simulink model "f7_VPP_DER_demo"  (R2019b)
settings: Solver=VariableStepAuto  StartTime=0.0  StopTime=2  FixedStep=1e-9  RelTol=1e-2
PreLoadFcn:
  | ss=2;sr=0;
InitFcn:
  | ss=2;sr=0;
libraries: powerlib x35, powerlib_meascontrol x30
settings Model: SimulationMode=accelerator  Creator=MAHMUD  LastModifiedBy=MAHMUD
settings SolverCC: ZeroCrossAlgorithm=Adaptive
settings DataIOCC: ReturnWorkspaceOutputs=off
settings DebuggingCC: MaxConsecutiveZCsMsg=none  IgnoredZcDiagnostic=none  ArithmeticOperatorsInVariantConditions=warning
settings SFSimCC: SimUseLocalCustomCode=off  CustomCodeUndefinedFunction=UseInterfaceOnly
settings RTWCC: RTWUseLocalCustomCode=off

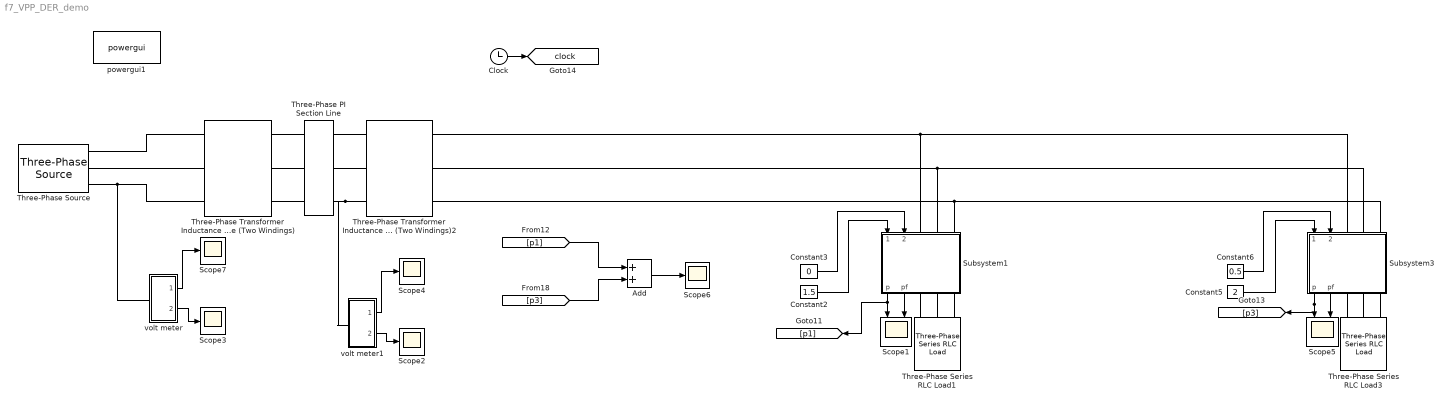
== system f7_VPP_DER_demo ==
  Add : Sum  Inputs=2
  Clock : Clock
  Constant2 : Constant  Value=1.5
  Constant3 : Constant  Value=0
  Constant5 : Constant  Value=2
  Constant6 : Constant  Value=0.5
  Scope1 : Scope  NumInputPorts=2
  Scope{2..4,6..7} (5 alike) : Scope
  Scope5 : Scope  NumInputPorts=2
  Subsystem1 : Subsystem
  Subsystem3 : Subsystem
  Three-Phase PI Section Line : powerlib/Elements/Three-Phase PI Section Line  LConnTagsString=a|b|c  RConnTagsString=A|B|C  Frequency=50  Resistances=[ 0.01273 0.3864]  Inductances="[ 0.9337e-3  4.1264e-3]"  Capacitances=[12.74e-9 7.751e-9]  Length=100
      settings: SourceProductName=Simscape Electrical
  Three-Phase Series RLC Load1 : powerlib/Elements/Three-Phase Series RLC Load  LConnTagsString=A|B|C  Configuration=Y (grounded)  NominalVoltage=240  Vabc=[240 240 240]  Vabcp=[1e3 1e3 1e3]  NominalFrequency=50  UnbalancedPower=off  ActivePower=5e3  InductivePower=0  CapacitivePower=0  Pabc=[10e3 9e3 11e3]  QLabc=[100 90 110]  QCabc=[100 90 110]  Pabcp=[10e3 9e3 11e3]  QLabcp=[100 90 110]  QCabcp=[100 90 110]  Measurements=None  LoadType=constant PQ
      settings: SourceProductName=Simscape Electrical
  Three-Phase Series RLC Load3 : powerlib/Elements/Three-Phase Series RLC Load  LConnTagsString=A|B|C  Configuration=Y (grounded)  NominalVoltage=240  Vabc=[1e3 1e3 1e3]  Vabcp=[1e3 1e3 1e3]  NominalFrequency=50  UnbalancedPower=off  ActivePower=2e3  InductivePower=5e3  CapacitivePower=0  Pabc=[10e3 9e3 11e3]  QLabc=[100 90 110]  QCabc=[100 90 110]  Pabcp=[10e3 9e3 11e3]  QLabcp=[100 90 110]  QCabcp=[100 90 110]  Measurements=None  LoadType=constant PQ
      settings: SourceProductName=Simscape Electrical
  Three-Phase Source : powerlib/Electrical Sources/Three-Phase Source  InternalConnection=Yg  VoltagePhases=off  Voltage=14270  PhaseAngle=0  Voltage_phases=[25e3 25e3 25e3]/sqrt(3)  PhaseAngles_phases=[0 -120 +120]  Frequency=50  NonIdealSource=on  SpecifyImpedance=off  Resistance=0.8929  Inductance=0  ShortCircuitLevel=100e6  BaseVoltage=15000  XRratio=7  BusType=PQ  Pref=30e3  Qref=0  Prefabc=[10e3, 10e3, 10e3]  Qrefabc=[0, 0, 0]  Qmin=-inf  Qmax=inf
      settings: SourceProductName=Simscape Electrical
  Three-Phase Transformer Inductance Matrix Type (Two Windings) : powerlib/Elements/Three-Phase Transformer Inductance Matrix Type (Two Windings)  CoreType=Three-limb or five-limb core  Winding1Connection=Yg  Winding2Connection=Yg  AutoTransformer=off  Measurements=None  NominalPower=[100e3, 50]  VLLnom=[25000, 130000]  WindingResistances=[0.01, 0.01]  NoLoadIexcPos=2  NoLoadPlossPos=1000  ShortCircuitReactancePos=0.06  ShortCircuitReactancePosAuto=0.06  NoLoadIexcZero=100  NoLoadPlossZero=1500  ShortCircuitReactanceZero=0.03  ShortCircuitReactanceZeroAuto=0.03
      settings: SourceProductName=Simscape Electrical  SourceProductBaseCode=PS
  Three-Phase Transformer Inductance Matrix Type (Two Windings)2 : powerlib/Elements/Three-Phase Transformer Inductance Matrix Type (Two Windings)  CoreType=Three-limb or five-limb core  Winding1Connection=Yg  Winding2Connection=Yg  AutoTransformer=off  Measurements=None  NominalPower=[30e3, 50]  VLLnom=[12700, 240]  WindingResistances=[0.01, 0.01]  NoLoadIexcPos=4  NoLoadPlossPos=1000  ShortCircuitReactancePos=0.06  ShortCircuitReactancePosAuto=0.06  NoLoadIexcZero=100  NoLoadPlossZero=1500  ShortCircuitReactanceZero=0.03  ShortCircuitReactanceZeroAuto=0.03
      settings: SourceProductName=Simscape Electrical  SourceProductBaseCode=PS
  powergui1 : powerlib/powergui  Priority=1  SimulationMode=Continuous  SampleTime=50e-6  frequency=60  Iterations=50  frequencyindice=50  Pbase=100e6  ErrMax=1e-4  UnitsV=kV  UnitsW=MW  buscounter=0  FunctionMessages=off  echomessages=off  EnableUseOfTLC=off  CurrentSourceSwitches=off  DisableSnubberDevices=off  DisableRonSwitches=off  DisableVfSwitches=off  DisplayEquations=off  AutomaticDiscreteSolvers=off  SolverType=Tustin/Backward Euler (TBE)  Interpol=off  ExternalGateDelay=off  methode=off  Ts=100  x0status=blocks  SPID=on  SwTol=0  HookPort=off  NonlinearTolerance=1e-4  nMaxIteration=100  ContinueOnMaxIteration=off  RestoreLinks=warning  ResistiveCurrentMeasurement=off  Frange=[0:2:500]  Ylog=off  Xlog=on  ShowGrid=off  save=off  variable=ZData  structure=0  ZoomFFT=off  StartTime=0.0  cycles=1  DisplayStyle=1  fundamental=60  FreqAxis=off  MaxFrequency=1000  frequencyindicesteady=1  RmsSteady=1  display=off
      settings: SourceProductName=Simscape Electrical
  volt meter : Subsystem
  volt meter1 : Subsystem
  tag scope: clock=global
  wires:
  Subsystem3/2(pf) -> Scope5/2
  Constant2/1 -> Subsystem1/1(stop time)
  volt meter1/2(Vrms) -> Scope2/1
  [p1] -> Add/1
  Constant3/1 -> Subsystem1/2(start time)
  Subsystem1/1(p) -> [p1], Scope1/1
  Subsystem1/2(pf) -> Scope1/2
  volt meter/1(Vsin) -> Scope7/1
  volt meter1/1(Vsin) -> Scope4/1
  volt meter/2(Vrms) -> Scope3/1
  Constant5/1 -> Subsystem3/1(stop time)
  Subsystem3/1(p) -> [p3], Scope5/1
  Constant6/1 -> Subsystem3/2(start time)
  [p3] -> Add/2
  Clock/1 -> [clock]
  Add/1 -> Scope6/1
  connections:
  Subsystem1/LConn2 -- Three-Phase Transformer Inductance Matrix Type (Two Windings)2/RConn2 -- Subsystem3/LConn2
  Three-Phase Transformer Inductance Matrix Type (Two Windings)/LConn3 -- Three-Phase Source/RConn3 -- volt meter/LConn1
  Subsystem1/LConn3 -- Three-Phase Transformer Inductance Matrix Type (Two Windings)2/RConn3 -- Subsystem3/LConn3
  Subsystem1/LConn1 -- Three-Phase Transformer Inductance Matrix Type (Two Windings)2/RConn1 -- Subsystem3/LConn1
  Three-Phase Transformer Inductance Matrix Type (Two Windings)2/LConn3 -- Three-Phase PI Section Line/RConn3 -- volt meter1/LConn1
  Subsystem3/RConn3 -- Three-Phase Series RLC Load3/LConn3
  Three-Phase Transformer Inductance Matrix Type (Two Windings)/RConn3 -- Three-Phase PI Section Line/LConn3
  Subsystem3/RConn1 -- Three-Phase Series RLC Load3/LConn1
  Three-Phase PI Section Line/RConn2 -- Three-Phase Transformer Inductance Matrix Type (Two Windings)2/LConn2
  Three-Phase PI Section Line/LConn1 -- Three-Phase Transformer Inductance Matrix Type (Two Windings)/RConn1
  Three-Phase Source/RConn1 -- Three-Phase Transformer Inductance Matrix Type (Two Windings)/LConn1
  Subsystem1/RConn2 -- Three-Phase Series RLC Load1/LConn2
  Subsystem1/RConn3 -- Three-Phase Series RLC Load1/LConn3
  Three-Phase PI Section Line/LConn2 -- Three-Phase Transformer Inductance Matrix Type (Two Windings)/RConn2
  Subsystem1/RConn1 -- Three-Phase Series RLC Load1/LConn1
  Three-Phase Source/RConn2 -- Three-Phase Transformer Inductance Matrix Type (Two Windings)/LConn2
  Three-Phase Transformer Inductance Matrix Type (Two Windings)2/LConn1 -- Three-Phase PI Section Line/RConn1
  Subsystem3/RConn2 -- Three-Phase Series RLC Load3/LConn2

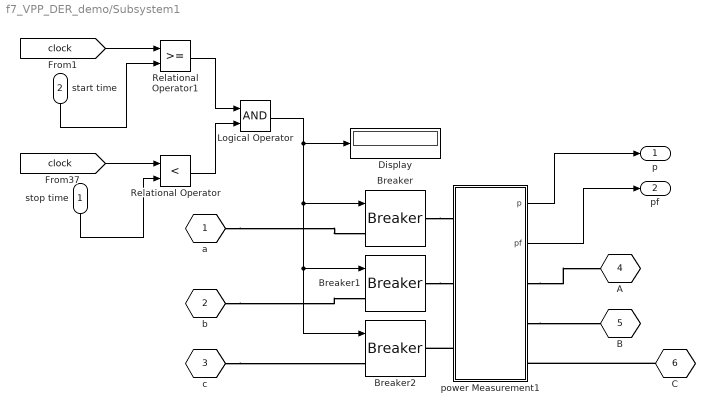
== system f7_VPP_DER_demo/Subsystem1 ==
  stop time : Inport
  start time : Inport  Port=2
  Breaker : powerlib/Elements/Breaker  InitialState=0  SwitchingTimes="[1/60  5/60]"  External=on  BreakerResistance=0.01  SnubberResistance=1e6  SnubberCapacitance=inf  Measurements=None  MoreParameters=on  NoBreakLoop=off
      settings: SourceProductName=Simscape Electrical
  Breaker1 : powerlib/Elements/Breaker  InitialState=0  SwitchingTimes="[1/60  5/60]"  External=on  BreakerResistance=0.01  SnubberResistance=1e6  SnubberCapacitance=inf  Measurements=None  MoreParameters=on  NoBreakLoop=off
      settings: SourceProductName=Simscape Electrical
  Breaker2 : powerlib/Elements/Breaker  InitialState=0  SwitchingTimes="[1/60  5/60]"  External=on  BreakerResistance=0.01  SnubberResistance=1e6  SnubberCapacitance=inf  Measurements=None  MoreParameters=on  NoBreakLoop=off
      settings: SourceProductName=Simscape Electrical
  Display : Display
  Logical Operator : Logic  AllPortsSameDT=off  OutDataTypeStr=boolean
  Relational Operator : RelationalOperator  Operator=<  OutDataTypeStr=boolean  ZeroCross=off  RndMeth=Simplest
  Relational Operator1 : RelationalOperator  OutDataTypeStr=boolean  ZeroCross=off  RndMeth=Simplest
  power Measurement1 : Subsystem
  a : PMIOPort  Tag=PMCPort  Side=Left
  b : PMIOPort  Tag=PMCPort  Port=2  Side=Left
  c : PMIOPort  Tag=PMCPort  Port=3  Side=Left
  "A " : PMIOPort  Tag=PMCPort  Port=4  Side=Right
  B : PMIOPort  Tag=PMCPort  Port=5  Side=Right
  C : PMIOPort  Tag=PMCPort  Port=6  Side=Right
  p : Outport
  pf : Outport  Port=2
  wires:
  Logical Operator/1 -> Breaker/1, Breaker2/1, Breaker1/1, Display/1
  [clock] -> Relational Operator/1
  stop time/1 -> Relational Operator/2
  [clock] -> Relational Operator1/1
  start time/1 -> Relational Operator1/2
  Relational Operator1/1 -> Logical Operator/1
  Relational Operator/1 -> Logical Operator/2
  power Measurement1/2(pf) -> pf/1
  power Measurement1/1(p) -> p/1
  connections:
  b/RConn1 -- Breaker1/LConn1
  c/RConn1 -- Breaker2/LConn1
  a/RConn1 -- Breaker/LConn1
  power Measurement1/RConn2 -- B/RConn1
  power Measurement1/LConn3 -- Breaker2/RConn1
  Breaker1/RConn1 -- power Measurement1/LConn2
  Breaker/RConn1 -- power Measurement1/LConn1
  C/RConn1 -- power Measurement1/RConn3
  power Measurement1/RConn1 -- "A "/RConn1

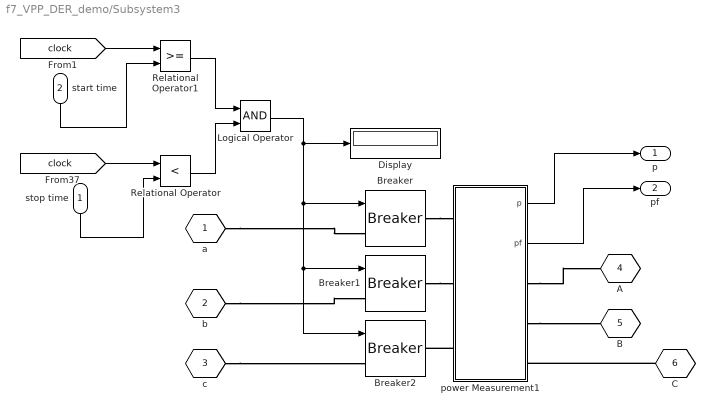
== system f7_VPP_DER_demo/Subsystem3 ==
  stop time : Inport
  start time : Inport  Port=2
  Breaker : powerlib/Elements/Breaker  InitialState=0  SwitchingTimes="[1/60  5/60]"  External=on  BreakerResistance=0.01  SnubberResistance=1e6  SnubberCapacitance=inf  Measurements=None  MoreParameters=on  NoBreakLoop=off
      settings: SourceProductName=Simscape Electrical
  Breaker1 : powerlib/Elements/Breaker  InitialState=0  SwitchingTimes="[1/60  5/60]"  External=on  BreakerResistance=0.01  SnubberResistance=1e6  SnubberCapacitance=inf  Measurements=None  MoreParameters=on  NoBreakLoop=off
      settings: SourceProductName=Simscape Electrical
  Breaker2 : powerlib/Elements/Breaker  InitialState=0  SwitchingTimes="[1/60  5/60]"  External=on  BreakerResistance=0.01  SnubberResistance=1e6  SnubberCapacitance=inf  Measurements=None  MoreParameters=on  NoBreakLoop=off
      settings: SourceProductName=Simscape Electrical
  Display : Display
  Logical Operator : Logic  AllPortsSameDT=off  OutDataTypeStr=boolean
  Relational Operator : RelationalOperator  Operator=<  OutDataTypeStr=boolean  ZeroCross=off  RndMeth=Simplest
  Relational Operator1 : RelationalOperator  OutDataTypeStr=boolean  ZeroCross=off  RndMeth=Simplest
  power Measurement1 : Subsystem
  a : PMIOPort  Tag=PMCPort  Side=Left
  b : PMIOPort  Tag=PMCPort  Port=2  Side=Left
  c : PMIOPort  Tag=PMCPort  Port=3  Side=Left
  "A " : PMIOPort  Tag=PMCPort  Port=4  Side=Right
  B : PMIOPort  Tag=PMCPort  Port=5  Side=Right
  C : PMIOPort  Tag=PMCPort  Port=6  Side=Right
  p : Outport
  pf : Outport  Port=2
  wires:
  Logical Operator/1 -> Breaker/1, Breaker2/1, Breaker1/1, Display/1
  [clock] -> Relational Operator/1
  stop time/1 -> Relational Operator/2
  [clock] -> Relational Operator1/1
  start time/1 -> Relational Operator1/2
  Relational Operator1/1 -> Logical Operator/1
  Relational Operator/1 -> Logical Operator/2
  power Measurement1/2(pf) -> pf/1
  power Measurement1/1(p) -> p/1
  connections:
  b/RConn1 -- Breaker1/LConn1
  c/RConn1 -- Breaker2/LConn1
  a/RConn1 -- Breaker/LConn1
  power Measurement1/RConn2 -- B/RConn1
  power Measurement1/LConn3 -- Breaker2/RConn1
  Breaker1/RConn1 -- power Measurement1/LConn2
  Breaker/RConn1 -- power Measurement1/LConn1
  C/RConn1 -- power Measurement1/RConn3
  power Measurement1/RConn1 -- "A "/RConn1

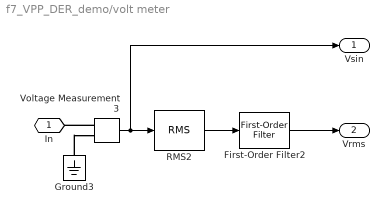
== system f7_VPP_DER_demo/volt meter ==
  First-Order Filter2 : powerlib_meascontrol/Filters/First-Order Filter  FilterType=Lowpass  Tc=100e-3  Ts=0  Initialize=off  Vac_Init=[0, 0, 50]  Vdc_Init=0  PlotResponse=off  FreqRange="[0,  200,  1]"
      settings: SourceProductName=Simscape Electrical
  Ground3 : powerlib/Elements/Ground  LConnTagsString=a
      settings: SourceProductName=Simscape Electrical
  RMS2 : powerlib_meascontrol/Measurements/RMS  TrueRMS=on  Freq=50  RMSInit=210  Ts=0.001
      settings: SourceProductName=Simscape Electrical
  Voltage Measurement3 : powerlib/Measurements/Voltage Measurement  PhasorSimulation=off  OutputType=Complex  PSBequivalent=0
      settings: SourceProductName=Simscape Electrical
  In : PMIOPort  Side=Left
  Vsin : Outport
  Vrms : Outport  Port=2
  wires:
  Voltage Measurement3/1 -> Vsin/1, RMS2/1
  RMS2/1 -> First-Order Filter2/1
  First-Order Filter2/1 -> Vrms/1
  connections:
  Ground3/LConn1 -- Voltage Measurement3/LConn2
  Voltage Measurement3/LConn1 -- In/RConn1

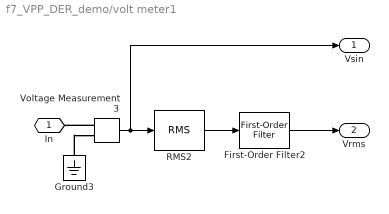
== system f7_VPP_DER_demo/volt meter1 ==
  First-Order Filter2 : powerlib_meascontrol/Filters/First-Order Filter  FilterType=Lowpass  Tc=100e-3  Ts=0  Initialize=off  Vac_Init=[0, 0, 50]  Vdc_Init=0  PlotResponse=off  FreqRange="[0,  200,  1]"
      settings: SourceProductName=Simscape Electrical
  Ground3 : powerlib/Elements/Ground  LConnTagsString=a
      settings: SourceProductName=Simscape Electrical
  RMS2 : powerlib_meascontrol/Measurements/RMS  TrueRMS=on  Freq=50  RMSInit=210  Ts=0.001
      settings: SourceProductName=Simscape Electrical
  Voltage Measurement3 : powerlib/Measurements/Voltage Measurement  PhasorSimulation=off  OutputType=Complex  PSBequivalent=0
      settings: SourceProductName=Simscape Electrical
  In : PMIOPort  Side=Left
  Vsin : Outport
  Vrms : Outport  Port=2
  wires:
  First-Order Filter2/1 -> Vrms/1
  RMS2/1 -> First-Order Filter2/1
  Voltage Measurement3/1 -> RMS2/1, Vsin/1
  connections:
  Voltage Measurement3/LConn1 -- In/RConn1
  Ground3/LConn1 -- Voltage Measurement3/LConn2

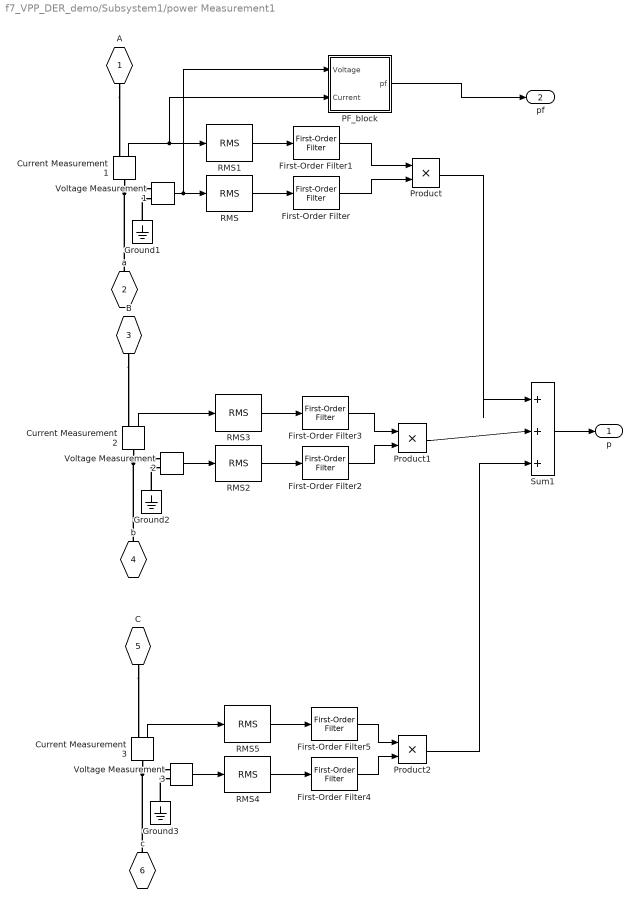
== system f7_VPP_DER_demo/Subsystem1/power Measurement1 ==
  Current Measurement1 : powerlib/Measurements/Current Measurement  PhasorSimulation=off  OutputType=Complex  PSBequivalent=0
      settings: SourceProductName=Simscape Electrical
  Current Measurement2 : powerlib/Measurements/Current Measurement  PhasorSimulation=off  OutputType=Complex  PSBequivalent=0
      settings: SourceProductName=Simscape Electrical
  Current Measurement3 : powerlib/Measurements/Current Measurement  PhasorSimulation=off  OutputType=Complex  PSBequivalent=0
      settings: SourceProductName=Simscape Electrical
  First-Order Filter{,1..5} (6 alike) : powerlib_meascontrol/Filters/First-Order Filter  FilterType=Lowpass  Tc=100e-3  Ts=0  Initialize=off  Vac_Init=[0, 0, 50]  Vdc_Init=0  PlotResponse=off  FreqRange="[0,  200,  1]"
      settings: SourceProductName=Simscape Electrical
  Ground1 : powerlib/Elements/Ground  LConnTagsString=a
      settings: SourceProductName=Simscape Electrical
  Ground2 : powerlib/Elements/Ground  LConnTagsString=a
      settings: SourceProductName=Simscape Electrical
  Ground3 : powerlib/Elements/Ground  LConnTagsString=a
      settings: SourceProductName=Simscape Electrical
  PF_block : Subsystem
  Product : Product
  Product1 : Product
  Product2 : Product
  RMS{,1..5} (6 alike) : powerlib_meascontrol/Measurements/RMS  TrueRMS=on  Freq=50  RMSInit=210  Ts=0.001
      settings: SourceProductName=Simscape Electrical
  Sum1 : Sum  Inputs=|+++
  Voltage Measurement1 : powerlib/Measurements/Voltage Measurement  PhasorSimulation=off  OutputType=Complex  PSBequivalent=0
      settings: SourceProductName=Simscape Electrical
  Voltage Measurement2 : powerlib/Measurements/Voltage Measurement  PhasorSimulation=off  OutputType=Complex  PSBequivalent=0
      settings: SourceProductName=Simscape Electrical
  Voltage Measurement3 : powerlib/Measurements/Voltage Measurement  PhasorSimulation=off  OutputType=Complex  PSBequivalent=0
      settings: SourceProductName=Simscape Electrical
  "A " : PMIOPort  Tag=PMCPort  Side=Right
  a : PMIOPort  Tag=PMCPort  Port=2  Side=Left
  B : PMIOPort  Tag=PMCPort  Port=3  Side=Right
  b : PMIOPort  Tag=PMCPort  Port=4  Side=Left
  C : PMIOPort  Tag=PMCPort  Port=5  Side=Right
  c : PMIOPort  Tag=PMCPort  Port=6  Side=Left
  p : Outport
  pf : Outport  Port=2
  wires:
  Current Measurement1/1 -> PF_block/2(Current), RMS1/1
  Sum1/1 -> p/1
  RMS/1 -> First-Order Filter/1
  RMS1/1 -> First-Order Filter1/1
  Voltage Measurement1/1 -> PF_block/1(Voltage), RMS/1
  First-Order Filter1/1 -> Product/1
  First-Order Filter/1 -> Product/2
  Product/1 -> Sum1/1
  Voltage Measurement2/1 -> RMS2/1
  RMS3/1 -> First-Order Filter3/1
  RMS2/1 -> First-Order Filter2/1
  Current Measurement2/1 -> RMS3/1
  Current Measurement3/1 -> RMS5/1
  RMS4/1 -> First-Order Filter4/1
  RMS5/1 -> First-Order Filter5/1
  Voltage Measurement3/1 -> RMS4/1
  First-Order Filter3/1 -> Product1/1
  First-Order Filter2/1 -> Product1/2
  First-Order Filter5/1 -> Product2/1
  First-Order Filter4/1 -> Product2/2
  Product1/1 -> Sum1/2
  Product2/1 -> Sum1/3
  PF_block/1(pf) -> pf/1
  connections:
  Ground1/LConn1 -- Voltage Measurement1/LConn2
  Current Measurement1/LConn1 -- a/RConn1 -- Voltage Measurement1/LConn1
  "A "/RConn1 -- Current Measurement1/RConn1
  b/RConn1 -- Current Measurement2/LConn1 -- Voltage Measurement2/LConn1
  B/RConn1 -- Current Measurement2/RConn1
  Ground2/LConn1 -- Voltage Measurement2/LConn2
  c/RConn1 -- Voltage Measurement3/LConn1 -- Current Measurement3/LConn1
  Ground3/LConn1 -- Voltage Measurement3/LConn2
  C/RConn1 -- Current Measurement3/RConn1

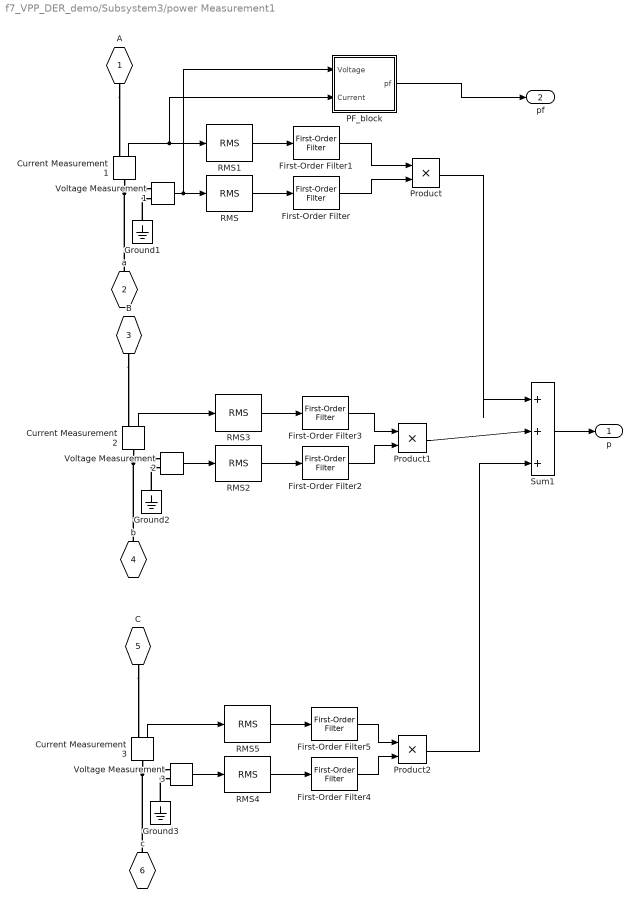
== system f7_VPP_DER_demo/Subsystem3/power Measurement1 ==
  Current Measurement1 : powerlib/Measurements/Current Measurement  PhasorSimulation=off  OutputType=Complex  PSBequivalent=0
      settings: SourceProductName=Simscape Electrical
  Current Measurement2 : powerlib/Measurements/Current Measurement  PhasorSimulation=off  OutputType=Complex  PSBequivalent=0
      settings: SourceProductName=Simscape Electrical
  Current Measurement3 : powerlib/Measurements/Current Measurement  PhasorSimulation=off  OutputType=Complex  PSBequivalent=0
      settings: SourceProductName=Simscape Electrical
  First-Order Filter{,1..5} (6 alike) : powerlib_meascontrol/Filters/First-Order Filter  FilterType=Lowpass  Tc=100e-3  Ts=0  Initialize=off  Vac_Init=[0, 0, 50]  Vdc_Init=0  PlotResponse=off  FreqRange="[0,  200,  1]"
      settings: SourceProductName=Simscape Electrical
  Ground1 : powerlib/Elements/Ground  LConnTagsString=a
      settings: SourceProductName=Simscape Electrical
  Ground2 : powerlib/Elements/Ground  LConnTagsString=a
      settings: SourceProductName=Simscape Electrical
  Ground3 : powerlib/Elements/Ground  LConnTagsString=a
      settings: SourceProductName=Simscape Electrical
  PF_block : Subsystem
  Product : Product
  Product1 : Product
  Product2 : Product
  RMS{,1..5} (6 alike) : powerlib_meascontrol/Measurements/RMS  TrueRMS=on  Freq=50  RMSInit=210  Ts=0.001
      settings: SourceProductName=Simscape Electrical
  Sum1 : Sum  Inputs=|+++
  Voltage Measurement1 : powerlib/Measurements/Voltage Measurement  PhasorSimulation=off  OutputType=Complex  PSBequivalent=0
      settings: SourceProductName=Simscape Electrical
  Voltage Measurement2 : powerlib/Measurements/Voltage Measurement  PhasorSimulation=off  OutputType=Complex  PSBequivalent=0
      settings: SourceProductName=Simscape Electrical
  Voltage Measurement3 : powerlib/Measurements/Voltage Measurement  PhasorSimulation=off  OutputType=Complex  PSBequivalent=0
      settings: SourceProductName=Simscape Electrical
  "A " : PMIOPort  Tag=PMCPort  Side=Right
  a : PMIOPort  Tag=PMCPort  Port=2  Side=Left
  B : PMIOPort  Tag=PMCPort  Port=3  Side=Right
  b : PMIOPort  Tag=PMCPort  Port=4  Side=Left
  C : PMIOPort  Tag=PMCPort  Port=5  Side=Right
  c : PMIOPort  Tag=PMCPort  Port=6  Side=Left
  p : Outport
  pf : Outport  Port=2
  wires:
  Current Measurement1/1 -> PF_block/2(Current), RMS1/1
  Sum1/1 -> p/1
  RMS/1 -> First-Order Filter/1
  RMS1/1 -> First-Order Filter1/1
  Voltage Measurement1/1 -> PF_block/1(Voltage), RMS/1
  First-Order Filter1/1 -> Product/1
  First-Order Filter/1 -> Product/2
  Product/1 -> Sum1/1
  Voltage Measurement2/1 -> RMS2/1
  RMS3/1 -> First-Order Filter3/1
  RMS2/1 -> First-Order Filter2/1
  Current Measurement2/1 -> RMS3/1
  Current Measurement3/1 -> RMS5/1
  RMS4/1 -> First-Order Filter4/1
  RMS5/1 -> First-Order Filter5/1
  Voltage Measurement3/1 -> RMS4/1
  First-Order Filter3/1 -> Product1/1
  First-Order Filter2/1 -> Product1/2
  First-Order Filter5/1 -> Product2/1
  First-Order Filter4/1 -> Product2/2
  Product1/1 -> Sum1/2
  Product2/1 -> Sum1/3
  PF_block/1(pf) -> pf/1
  connections:
  Ground1/LConn1 -- Voltage Measurement1/LConn2
  Current Measurement1/LConn1 -- a/RConn1 -- Voltage Measurement1/LConn1
  "A "/RConn1 -- Current Measurement1/RConn1
  b/RConn1 -- Current Measurement2/LConn1 -- Voltage Measurement2/LConn1
  B/RConn1 -- Current Measurement2/RConn1
  Ground2/LConn1 -- Voltage Measurement2/LConn2
  c/RConn1 -- Voltage Measurement3/LConn1 -- Current Measurement3/LConn1
  Ground3/LConn1 -- Voltage Measurement3/LConn2
  C/RConn1 -- Current Measurement3/RConn1

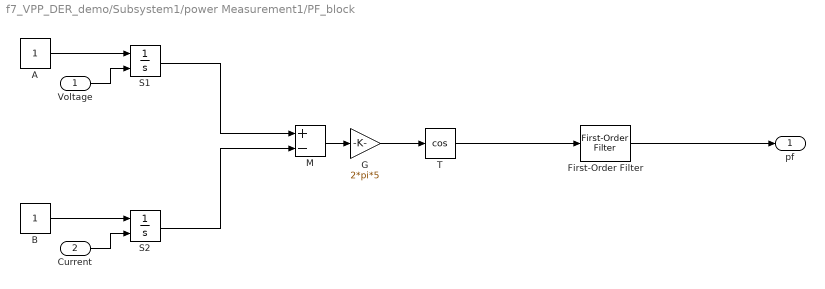
== system f7_VPP_DER_demo/Subsystem1/power Measurement1/PF_block ==
  Voltage : Inport
  Current : Inport  Port=2
  A : Constant
  B : Constant
  First-Order Filter : powerlib_meascontrol/Filters/First-Order Filter  FilterType=Lowpass  Tc=100e-3  Ts=0  Initialize=off  Vac_Init=[0, 0, 50]  Vdc_Init=0  PlotResponse=off  FreqRange="[0,  200,  1]"
      settings: SourceProductName=Simscape Electrical
  G : Gain  Gain=2*pi*5
  M : Sum  Inputs=+-
  S1 : Integrator  ExternalReset=falling  ZeroCross=off
  S2 : Integrator  ExternalReset=falling  ZeroCross=off
  T : Trigonometry  Operator=cos
  pf : Outport
  wires:
  M/1 -> G/1
  Voltage/1 -> S1/2
  S2/1 -> M/2
  A/1 -> S1/1
  S1/1 -> M/1
  Current/1 -> S2/2
  G/1 -> T/1
  B/1 -> S2/1
  First-Order Filter/1 -> pf/1
  T/1 -> First-Order Filter/1

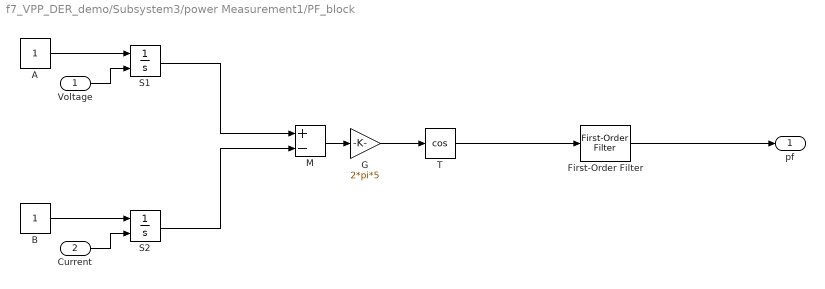
== system f7_VPP_DER_demo/Subsystem3/power Measurement1/PF_block ==
  Voltage : Inport
  Current : Inport  Port=2
  A : Constant
  B : Constant
  First-Order Filter : powerlib_meascontrol/Filters/First-Order Filter  FilterType=Lowpass  Tc=100e-3  Ts=0  Initialize=off  Vac_Init=[0, 0, 50]  Vdc_Init=0  PlotResponse=off  FreqRange="[0,  200,  1]"
      settings: SourceProductName=Simscape Electrical
  G : Gain  Gain=2*pi*5
  M : Sum  Inputs=+-
  S1 : Integrator  ExternalReset=falling  ZeroCross=off
  S2 : Integrator  ExternalReset=falling  ZeroCross=off
  T : Trigonometry  Operator=cos
  pf : Outport
  wires:
  M/1 -> G/1
  Voltage/1 -> S1/2
  S2/1 -> M/2
  A/1 -> S1/1
  S1/1 -> M/1
  Current/1 -> S2/2
  G/1 -> T/1
  B/1 -> S2/1
  First-Order Filter/1 -> pf/1
  T/1 -> First-Order Filter/1
